simulink model "BD_PAR_AUTO_base_model"  (Simulink 10.3)
settings: Solver=ode1  StartTime=0.0  StopTime=max(cyc_mph(:,1))  FixedStep=1  MaxStep=1  RelTol=1e-3  AbsTol=1e-3
undefined symbols (not defined in the file): acc_dcdc_eff, acc_elec_eff, acc_elec_pwr, acc_mech_eff, acc_mech_pwr, acc_mech_trq, air_cp, amb_tmp, cs_charge_deplete_bool, cs_charge_trq, cs_electric_decel_spd, cs_electric_launch_spd_hi, cs_electric_launch_spd_lo, cs_hi_soc, cs_lo_soc, cs_min_trq_frac, cs_off_trq_frac, cyc_avg_time, cyc_cargo_mass, cyc_elevation_init, cyc_filter_bool, cyc_grade, cyc_mph, enable_sim_stop_distance, enable_sim_stop_max_spd, enable_sim_stop_speed, enable_sim_stop_time, enable_stop, enable_stop_fc, ess_cap_scale, ess_coulombic_eff, ess_init_soc, ess_max_ah_cap, ess_max_volts, ess_min_volts, ess_mod_airflow, ess_mod_cp, ess_mod_init_tmp, ess_module_mass, ess_module_num, ess_on, ess_r_chg, ess_r_dis, ess_res_scale_coef, ess_res_scale_fun, ess_set_tmp, ess_soc, ess_th_calc, ess_th_res_off, ess_th_res_on, ess_tmp, ess_voc, ex_calc, ex_cat_co_frac, ex_cat_ext_cp, ex_cat_ext_emisv, ex_cat_ext_init_tmp, ex_cat_ext_mass, ex_cat_ext_sarea, ex_cat_hc_frac ... (+168)
(part 3 of 15)

== system BD_PAR_AUTO_base_model/<vc> par auto/motor controller logic ==
  bus voltage : Inport
  req'd input power (W) : Inport  Port=2
  req'd output spd (rad/s) : Inport  Port=3
  shifting : Inport  Port=4
  Abs : Abs
  Abs1 : Abs
  Block NOTES : Subsystem
      mask Display: disp('Block\nNOTES')
  Constant : Constant  Value=mc_max_crrnt
  Constant1 : Constant  Value=0.001
  Constant2 : Constant  Value=0
  Logical Operator1 : Logic  Operator=NOT  Inputs=1
  Memory : Memory  InitialCondition=ess_module_num*mean(ess_voc(1,:))
  MinMax : MinMax  Inputs=2  InputSameDT=on  SaturateOnIntegerOverflow=on
  Product1 : Product  InputSameDT=on  RndMeth=Zero  SaturateOnIntegerOverflow=on  OutDataTypeStr=Inherit: Same as first input
  Relational Operator : RelationalOperator  Operator=<=  RndMeth=Nearest  InputSameDT=on
  Relational Operator2 : RelationalOperator  Operator===  RndMeth=Nearest  InputSameDT=on
  Sign : Subsystem  mask(Sign){}
      mask help: y = sign(x)
      mask Help: Sign Function:\n\t\t\ty = 1 if x > 0\n\t\t\ty = 0 if x = 0\n\t\t\ty = -1 if x < 0
      mask Display: plot(-50,-50,50,50,[-50,50],[0,0],[0,0],[-50,50],[-40,0],[-30,-30],[0,40],[30,30])
  Switch : Switch  Threshold=eps
  current-limited power : Product  InputSameDT=on  RndMeth=Zero  SaturateOnIntegerOverflow=on  OutDataTypeStr=Inherit: Same as first input
  true if motor should be shut down : Logic  Operator=OR
  req'd input power (W)1 : Outport  InitialOutput=0
  tag scope: mc_crrnt_limited=global
  wires:
  shifting/1 -> true if motor should be shut down/2
  Logical Operator1/1 -> Switch/2
  true if motor should be shut down/1 -> Logical Operator1/1
  Memory/1 -> Product1/1
  bus voltage/1 -> Memory/1
  Constant/1 -> Product1/2
  req'd input power (W)/1 -> Abs/1, Sign/1(in_1)
  Abs/1 -> MinMax/2
  Sign/1(out_1) -> current-limited power/2
  Constant2/1 -> Switch/3
  Switch/1 -> req'd input power (W)1/1
  current-limited power/1 -> Switch/1
  Product1/1 -> MinMax/1, Relational Operator2/1
  MinMax/1 -> current-limited power/1, Relational Operator2/2
  Relational Operator2/1 -> [mc_crrnt_limited]
  Relational Operator/1 -> true if motor should be shut down/1
  Constant1/1 -> Relational Operator/2
  req'd output spd (rad/s)/1 -> Abs1/1
  Abs1/1 -> Relational Operator/1

== system BD_PAR_AUTO_base_model/<vc> par auto/parallel clutch control ==
  shifting : Inport
  gb_trq_in_r : Inport  Port=2
  gb_spd_in_r : Inport  Port=3
  engine on : Inport  Port=4
  Block NOTES : Subsystem
      mask Display: disp('Block\nNOTES')
  Clock : Clock
  Constant : Constant  Value=1e-3
  Constant1 : Constant  Value=vc_clutch_bool
  Constant2 : Constant  Value=vc_idle_spd
  Constant3 : Constant  Value=1e-3
  Constant4 : Constant  Value=vc_launch_spd
  Constant5 : Constant  Value=2.5
  Constant6 : Constant
  Fcn: 1 if clutch disengaged 2 if clutch slipping 3 if clutch engaged : Fcn  Expr=u[1]+2*u[2]*(1-u[1])*(1-u[3])+3*u[3]*(1-u[1])
  Logical Operator : Logic
  Logical Operator1 : Logic  Operator=OR
  Manual Switch : ManualSwitch
  Memory : Memory  InitialCondition=1+(2*(cyc_mph(1,2)>0))
  Memory1 : Memory  InitialCondition=cyc_mph(1,2)>0
  Memory2 : Memory  InitialCondition=-1
  Mux : Mux  Inputs=3
  Relational Operator : RelationalOperator  Operator=<=  RndMeth=Nearest  InputSameDT=on
  Relational Operator1 : RelationalOperator  Operator=<  RndMeth=Nearest  InputSameDT=on
  Relational Operator2 : RelationalOperator  Operator=>  RndMeth=Nearest  InputSameDT=on
  Relational Operator3 : RelationalOperator  Operator=<  RndMeth=Nearest  InputSameDT=on
  Sum : Sum  Inputs=+-  InputSameDT=on  SaturateOnIntegerOverflow=on  OutDataTypeStr=Inherit: Same as first input
  Switch : Switch  Threshold=eps
  Switch1 : Switch  Threshold=0.5
  Transport Delay : TransportDelay  DelayTime=0.2
  clutch disengaged : Logic  Operator=OR
  clutch engaged : Logic  Operator=NOR
  clutch slipping : Logic  Inputs=3
  clutch slipping1 : Logic
  clutch slipping2 : Logic
  clutch was NOT fully engaged during last time step : RelationalOperator  Operator=<  RndMeth=Nearest  InputSameDT=on
  gearbox speed estimator : Subsystem
  clutch state : Outport
  wires:
  Switch/1 -> Memory/1, clutch state/1
  Fcn: 1 if clutch disengaged 2 if clutch slipping 3 if clutch engaged/1 -> Switch/1
  Manual Switch/1 -> Switch/2
  Switch1/1 -> Manual Switch/2
  gearbox speed estimator/1(Out1) -> Relational Operator3/1, Relational Operator1/1
  gb_spd_in_r/1 -> gearbox speed estimator/1(gb_spd_in_r if no gear change)
  Sum/1 -> Switch1/2
  Memory2/1 -> Sum/2
  Clock/1 -> Memory2/1, Sum/1
  clutch slipping2/1 -> Switch1/3
  Transport Delay/1 -> clutch slipping2/2
  clutch slipping1/1 -> Switch1/1
  Memory1/1 -> clutch slipping1/2
  engine on/1 -> Manual Switch/1, clutch slipping2/1, Transport Delay/1, Memory1/1, clutch slipping1/1
  Relational Operator1/1 -> Logical Operator1/2
  Constant2/1 -> Relational Operator1/2
  Mux/1 -> Fcn: 1 if clutch disengaged 2 if clutch slipping 3 if clutch engaged/1
  clutch engaged/1 -> Mux/3
  clutch disengaged/1 -> clutch engaged/1, Mux/1
  Constant3/1 -> Relational Operator2/2
  Relational Operator2/1 -> clutch slipping/1
  clutch slipping/1 -> clutch engaged/2, Mux/2
  Constant4/1 -> Relational Operator3/2
  Relational Operator3/1 -> clutch slipping/2
  Memory/1 -> clutch was NOT fully engaged during last time step/1
  Constant5/1 -> clutch was NOT fully engaged during last time step/2
  clutch was NOT fully engaged during last time step/1 -> clutch slipping/3
  Constant1/1 -> Logical Operator1/1
  Constant/1 -> Relational Operator/2
  Relational Operator/1 -> Logical Operator/1
  Logical Operator1/1 -> Logical Operator/2
  gb_trq_in_r/1 -> Relational Operator2/1, Relational Operator/1
  Logical Operator/1 -> clutch disengaged/2
  shifting/1 -> clutch disengaged/1
  Constant6/1 -> Switch/3

== system BD_PAR_AUTO_base_model/<vc> par auto/sim stop subsystem ==
  Block NOTES : Subsystem
      mask Display: disp('Block\nNOTES')
  Clock : Clock
  Logical Operator : Logic
  Product{,1..3} (4 alike) : Product  InputSameDT=on  RndMeth=Zero  SaturateOnIntegerOverflow=on  OutDataTypeStr=Inherit: Same as first input
  Relational Operator : RelationalOperator  Operator=>  RndMeth=Nearest  InputSameDT=on
  Relational Operator1 : RelationalOperator  Operator===  RndMeth=Nearest  InputSameDT=on
  Stop Simulation : Stop
  Stop Simulation1 : Stop
  Sum : Sum  Inputs=++++  InputSameDT=on  SaturateOnIntegerOverflow=on  OutDataTypeStr=Inherit: Same as first input
  Sum1 : Sum  Inputs=++++  InputSameDT=on  SaturateOnIntegerOverflow=on  OutDataTypeStr=Inherit: Same as first input
  do ex calcs?2 : Constant  Value=enable_stop_fc
  do ex calcs?3 : Constant  Value=enable_sim_stop_distance
  do ex calcs?4 : Constant  Value=enable_sim_stop_speed
  do ex calcs?5 : Constant  Value=enable_sim_stop_time
  do ex calcs?6 : Constant  Value=enable_sim_stop_max_spd
  do ex calcs?7 : Constant  Value=0
  stop sim distance : Subsystem  TreatAsAtomicUnit=on
  stop sim fc : Subsystem  TreatAsAtomicUnit=on
  stop sim max spd : Subsystem  TreatAsAtomicUnit=on
  stop sim speed : Subsystem  TreatAsAtomicUnit=on
  stop sim time : Subsystem  TreatAsAtomicUnit=on
  wires:
  do ex calcs?2/1 -> stop sim fc/Enable
  [engine_on] -> stop sim fc/1(engine on?)
  [distance] -> stop sim distance/1(distance)
  [mpha] -> stop sim speed/1(speed)
  Clock/1 -> stop sim time/1(time)
  [mpha] -> stop sim max spd/1(speed)
  stop sim distance/1(Out1) -> Product/2
  do ex calcs?3/1 -> stop sim distance/Enable, Product/1, Sum/1
  stop sim max spd/1(Out1) -> Product3/2
  stop sim time/1(Out1) -> Product2/2
  stop sim speed/1(Out1) -> Product1/2
  do ex calcs?4/1 -> stop sim speed/Enable, Product1/1, Sum/2
  do ex calcs?5/1 -> stop sim time/Enable, Product2/1, Sum/3
  do ex calcs?6/1 -> stop sim max spd/Enable, Product3/1, Sum/4
  Product/1 -> Sum1/1
  Product1/1 -> Sum1/2
  Product2/1 -> Sum1/3
  Product3/1 -> Sum1/4
  Logical Operator/1 -> Stop Simulation/1
  Sum1/1 -> Relational Operator1/2
  Sum/1 -> Relational Operator1/1, Relational Operator/1
  do ex calcs?7/1 -> Relational Operator/2
  Relational Operator/1 -> Logical Operator/1
  Relational Operator1/1 -> Logical Operator/2
  stop sim fc/1(Out1) -> Stop Simulation1/1

== system BD_PAR_AUTO_base_model/Interactive Graphics/off ==
  Altia_Run : Constant  Value=0
  tag scope: Altia_Run=global
  wires:
  Altia_Run/1 -> [Altia_Run]

== system BD_PAR_AUTO_base_model/NOTES/NOTES ==
  note: ADVISOR 2.0.2 10/7/98
      | Copyright 1998-2003  MRI, NREL.
      | All rights reserved
      |
      |  Notice:  This computer software was
      |  prepared by NREL/MRI, and hereinafter the Contractor,
      | under Contract No. DE-AC36-83CH10093 with
      | the Department of Energy (DOE).  All rights
      | in the computer software are reserved by DOE
      | on behalf of the United States Government and
      | the Contractor as provided in the contract.
      | You are authorized to use this computer software
      | for Governmental purposes but it is not to be
      | released or distributed to the public.  NEITHER
      | THE GOVERNMENT NOR THE CONTRACTOR MAKES ANY
      | WARRANTY, EXPRESS OR IMPLIED, OR ASSUMES ANY
      | LIABILITY FOR THE USE OF THIS SOFTWARE.
      | This notice including this sentence must
      | appear on any copies of this computer software.

== system BD_PAR_AUTO_base_model/clutch <cl>/help ==

== system BD_PAR_AUTO_base_model/drive cycle <cyc>/Block NOTES ==
  note: This block determines the speed required of the vehicle.  If cyc_filter_bool
      | is true, a centered-in-time average of the trace, with backlash, is required of
      | the vehicle.  This may be useful to smooth out jumps in the trace.  Otherwise,
      | the trace, exactly as published, is required of the vehicle.
      | This block also determines the roadway grade of the cycle and the
      | elevation as a function of the distance travelelled

== system BD_PAR_AUTO_base_model/drive cycle <cyc>/ambient pressure calc (atm) ==
  elevation : Inport
  Gain1 : Gain  Gain=-1  SaturateOnIntegerOverflow=on  OutDataTypeStr=Inherit: Same as input  ParamDataTypeStr=Inherit: Same as input
  Height Scale Factor (1/m) : Constant  Value=1.16546e-4
  Math Function : Math  SignedPower=on
  Product9 : Product  InputSameDT=on  RndMeth=Zero  SaturateOnIntegerOverflow=on  OutDataTypeStr=Inherit: Same as first input
  Out1 : Outport
  wires:
  Math Function/1 -> Out1/1
  Height Scale Factor (1/m)/1 -> Product9/2
  Gain1/1 -> Product9/1
  elevation/1 -> Gain1/1
  Product9/1 -> Math Function/1

== system BD_PAR_AUTO_base_model/drive cycle <cyc>/distance travelled (m) ==
  Block NOTES : Subsystem
      mask Display: disp('Block\nNOTES')
  Integrator : Integrator
  mph-->m/s : Gain  Gain=0.447  SaturateOnIntegerOverflow=on  OutDataTypeStr=Inherit: Same as input  ParamDataTypeStr=Inherit: Same as input
  Out1 : Outport  InitialOutput=0
  wires:
  mph-->m/s/1 -> Integrator/1
  [mpha] -> mph-->m/s/1
  Integrator/1 -> Out1/1

== system BD_PAR_AUTO_base_model/drive cycle <cyc>/repeated cycle grade vs. distance ==
  distance travelled (m) : Inport
  Fcn1 : Fcn  Expr=rem(u[1],period)
  Look-Up Table : Lookup  InputValues=t  Table=y
  out_1 : Outport  InitialOutput=0
  wires:
  Look-Up Table/1 -> out_1/1
  Fcn1/1 -> Look-Up Table/1
  distance travelled (m)/1 -> Fcn1/1

== system BD_PAR_AUTO_base_model/drive cycle <cyc>/repeated cycle speed vs. time ==
  Clock : Clock
  Fcn1 : Fcn  Expr=rem(u[1],period)
  Look-Up Table : Lookup  InputValues=t  Table=y
  out_1 : Outport  InitialOutput=0
  wires:
  Look-Up Table/1 -> out_1/1
  Clock/1 -> Fcn1/1
  Fcn1/1 -> Look-Up Table/1

== system BD_PAR_AUTO_base_model/drive cycle <cyc>/repeated cycle vehicle cargo mass vs. distance ==
  distance travelled (m) : Inport
  Fcn1 : Fcn  Expr=rem(u[1],period)
  Look-Up Table : Lookup  InputValues=t  Table=y
  out_1 : Outport  InitialOutput=0
  wires:
  Look-Up Table/1 -> out_1/1
  Fcn1/1 -> Look-Up Table/1
  distance travelled (m)/1 -> Fcn1/1

== system BD_PAR_AUTO_base_model/drive cycle <cyc>/super-smooth, no-lag trace ==
  Subsystem : Subsystem  mask(Running Average){n=avgtime}
      mask prompts: n "Averaging Time (s)"
      mask help: Running Average
      mask Help: Output is the average of the last (Averaging Time) seconds of input.
      mask Display: disp('Running\nAverage')
  repeated cycle : Subsystem
  out_1 : Outport  InitialOutput=0
  wires:
  repeated cycle/1(out_1) -> Subsystem/1(in_1)
  Subsystem/1(out_1) -> out_1/1

== system BD_PAR_AUTO_base_model/electric acc loads <acc>/Electrical Accessory Loads v2 <acc> ==
  note: Data Logging
  note: Backward-Forward Models
  note: INTERFACE
  "requested electrical Power, out to the driveline (W)" : Inport
  achieved power in from power source (W) : Inport  Port=2
  on/off : Inport  Port=3
  Accessory SDO : Subsystem
  Block NOTES : Subsystem
      mask Display: disp('Block\nNOTES')
  Mux3 : Mux  Inputs=3
  backward model : Subsystem
  forward model : Subsystem
  memory : Memory  InitialCondition=acc_elec_pwr
  "requested electrical Power, in from the power source (W)" : Outport
  "achieved electrical Power, out to the driveline (W)" : Outport  Port=2
  tag scope: acc_elec_pwr_a=global, acc_elec_pwr_est=global, acc_elec_pwr_r=global
  wires:
  [acc_on] -> backward model/2(on/off)
  on/off/1 -> [acc_on]
  memory/1 -> [acc_elec_pwr_est]
  forward model/2(acc_pwr_out) -> memory/1, [acc_elec_pwr_a]
  [acc_elec_pwr_r] -> forward model/2(acc_pwr_in)
  [acc_elec_pwr_est] -> Mux3/3
  [acc_elec_pwr_a] -> Mux3/2
  [acc_elec_pwr_r] -> Mux3/1
  backward model/2(elec_acc_out) -> [acc_elec_pwr_r]
  Mux3/1 -> Accessory SDO/1(data bus)
  forward model/1(pwr_out) -> [driveline_pwr_out_a]
  [powersource_pwr_in_a] -> forward model/1(pwr_in)
  backward model/1(elec_out) -> [powersource_pwr_in_r]
  [driveline_pwr_out_r] -> backward model/1(pwr_in)
  [driveline_pwr_out_a] -> "achieved electrical Power, out to the driveline (W)"/1
  [powersource_pwr_in_r] -> "requested electrical Power, in from the power source (W)"/1
  achieved power in from power source (W)/1 -> [powersource_pwr_in_a]
  "requested electrical Power, out to the driveline (W)"/1 -> [driveline_pwr_out_r]

== system BD_PAR_AUTO_base_model/electric assist control strategy <cs>/chg trq req'd (Nm) ==
  Constant : Constant  Value=cs_charge_trq*fc_trq_scale
  Constant1 : Constant  Value=ess_on
  Goal : Constant  Value=(cs_lo_soc+cs_hi_soc)/2
  Product : Product  InputSameDT=on  RndMeth=Zero  SaturateOnIntegerOverflow=on  OutDataTypeStr=Inherit: Same as first input
  Product1 : Product  Inputs=*/  InputSameDT=on  RndMeth=Zero  SaturateOnIntegerOverflow=on  OutDataTypeStr=Inherit: Same as first input
  Range : Constant  Value=(cs_hi_soc-cs_lo_soc)/2
  Saturation : Saturate  UpperLimit=inf  LowerLimit=-inf
  Sum : Sum  Inputs=-+  InputSameDT=on  SaturateOnIntegerOverflow=on  OutDataTypeStr=Inherit: Same as first input
  Switch : Switch  Threshold=eps
  add'l trq req'd (Nm) : Outport
  wires:
  Constant1/1 -> Switch/3, Switch/2
  Switch/1 -> add'l trq req'd (Nm)/1
  Saturation/1 -> Switch/1
  [SOC] -> Sum/1
  Goal/1 -> Sum/2
  Range/1 -> Product1/2
  Sum/1 -> Product1/1
  Product1/1 -> Product/2
  Constant/1 -> Product/1
  Product/1 -> Saturation/1

== system BD_PAR_AUTO_base_model/electric assist control strategy <cs>/help ==

== system BD_PAR_AUTO_base_model/electric assist control strategy <cs>/minimum trq (Nm) ==
  "trq and spd req'd into trq coupler (N*m, rad/s)" : Inport
  (--) : Constant  Value=cs_lo_soc
  Constant : Constant  Value=0
  Gain : Gain  Gain=cs_min_trq_frac  SaturateOnIntegerOverflow=on  OutDataTypeStr=Inherit: Same as input  ParamDataTypeStr=Inherit: Same as input
  Relational Operator2 : RelationalOperator  Operator=<  RndMeth=Nearest  InputSameDT=on
  Selector : Selector  InputPortWidth=2  IndexOptions=Index vector (dialog)  Indices=2  OutputSizes=1
  Switch : Switch  Threshold=eps
  Terminator : Terminator
  constant threshhold trq (N*m) : Constant  Value=max(fc_max_trq)*0.33
  max_torque lookup : Lookup  InputValues=fc_map_spd  Table=fc_max_trq*fc_trq_scale
  minimum trq (N*m) : Outport
  wires:
  Gain/1 -> Switch/1
  max_torque lookup/1 -> Gain/1
  Selector/1 -> max_torque lookup/1
  "trq and spd req'd into trq coupler (N*m, rad/s)"/1 -> Selector/1
  constant threshhold trq (N*m)/1 -> Terminator/1
  Constant/1 -> Switch/3
  Switch/1 -> minimum trq (N*m)/1
  Relational Operator2/1 -> Switch/2
  (--)/1 -> Relational Operator2/2
  [SOC] -> Relational Operator2/1

== system BD_PAR_AUTO_base_model/energy storage <ess>/ess config ==
  power req'd into bus (W) : Inport
  energy storage <ess> : Subsystem
      mask Display: image(imread('bdi_ess.jpg'))
  power available to bus (W) : Outport
  wires:
  power req'd into bus (W)/1 -> energy storage <ess>/1(power req'd into bus (W))
  energy storage <ess>/1(power available to bus (W)) -> power available to bus (W)/1

== system BD_PAR_AUTO_base_model/exhaust sys <ex>/Block NOTES ==
  note: This block models the exhaust system of an internal combustion engine (ICE).  Emphasis is on the catalytic converter
      | aftertreatment of emissions.  Since converter performance is tied to operating temperature, the temperature and heat
      | flows of the exhaust gas, converter, and engine manifold/downpipe are predicted.

== system BD_PAR_AUTO_base_model/exhaust sys <ex>/ex gas heat flow ==
  emis cat'd : Inport
  ex gas flow : Inport  Port=2
  Tex,eo : Inport  Port=3
  ex_temp : Inport  Port=4
  Enable : EnablePort  StatesWhenEnabling=reset
  % : Gain  Gain=100  SaturateOnIntegerOverflow=on
  %1 : Gain  Gain=669  SaturateOnIntegerOverflow=on
  %2 : Gain  Gain=121  SaturateOnIntegerOverflow=on
  %3 : Gain  Gain=93+79/3  SaturateOnIntegerOverflow=on
  %5 : Gain  Gain=0  SaturateOnIntegerOverflow=on
  (eo-tp)/exg : Product  Inputs=*/  SaturateOnIntegerOverflow=on
  Block NOTES : Subsystem
      mask Display: disp('Block\nNOTES')
  Demux3 : Demux
  Memory : Memory  InitialCondition=[0 0 0 0]
  Mux17 : Mux
  Mux19 : Mux  Inputs=3
  Qcp5 : Sum  Inputs=+-  SaturateOnIntegerOverflow=on
  Saturation1 : Saturate  UpperLimit=1  LowerLimit=0
  converter : Subsystem
  cp,exg : Gain  Gain=ex_gas_cp/1000  SaturateOnIntegerOverflow=on
  dTcat : Sum  Inputs=++++  SaturateOnIntegerOverflow=on
  h,exg : Fcn  Expr=23*((u/10)^0.8)
  inlet pipe : Subsystem
  "manifold " : Subsystem
  mol_EO/s : Gain  Gain=[1/44.1 1/28 1/46 1/44]  SaturateOnIntegerOverflow=on
  mol_ex/s : Gain  Gain=1/29  SaturateOnIntegerOverflow=on
  tailpipe  emis : Product  SaturateOnIntegerOverflow=on
  Tex,gas : Outport  OutputWhenDisabled=reset  InitialOutput=amb_tmp
  Qcat : Outport  Port=2  OutputWhenDisabled=reset  InitialOutput=0
  Qex : Outport  Port=3  OutputWhenDisabled=reset  InitialOutput=0
  wires:
  Memory/1 -> mol_EO/s/1
  emis cat'd/1 -> Memory/1
  ex gas flow/1 -> cp,exg/1, h,exg/1, mol_ex/s/1
  "manifold "/1(Texgo) -> inlet pipe/3(Texgi)
  %2/1 -> dTcat/3
  %3/1 -> dTcat/2
  %1/1 -> dTcat/1
  dTcat/1 -> tailpipe  emis/1
  tailpipe  emis/1 -> Qcat/1
  Mux19/1 -> Tex,gas/1
  Mux17/1 -> Qex/1
  [Tgmo] -> Mux19/3
  [Tgpo] -> Mux19/2
  converter/1(Texgo) -> Mux19/1
  converter/2(Qcm2g) -> Mux17/1
  converter/3(Qci2g) -> Mux17/2
  [Qp2g] -> Mux17/3
  [Qma2g] -> Mux17/4
  %5/1 -> dTcat/4
  inlet pipe/1(Texgo) -> converter/3(Texgi)
  Demux3/2 -> Qcp5/1
  Demux3/3 -> Qcp5/2, %2/1
  Demux3/1 -> %1/1
  Qcp5/1 -> %3/1
  Demux3/4 -> %5/1
  Saturation1/1 -> %/1
  mol_ex/s/1 -> (eo-tp)/exg/2
  mol_EO/s/1 -> (eo-tp)/exg/1
  (eo-tp)/exg/1 -> Saturation1/1
  Tex,eo/1 -> "manifold "/3(Texgi)
  ex_temp/1 -> inlet pipe/4(Tex), converter/4(Tex), "manifold "/4(Tex)
  cp,exg/1 -> inlet pipe/2(Cexg), tailpipe  emis/2, converter/2(Cexg), "manifold "/2(Cexg)
  h,exg/1 -> inlet pipe/1(h,exg), converter/1(h,exg), "manifold "/1(h,exg)
  %/1 -> Demux3/1

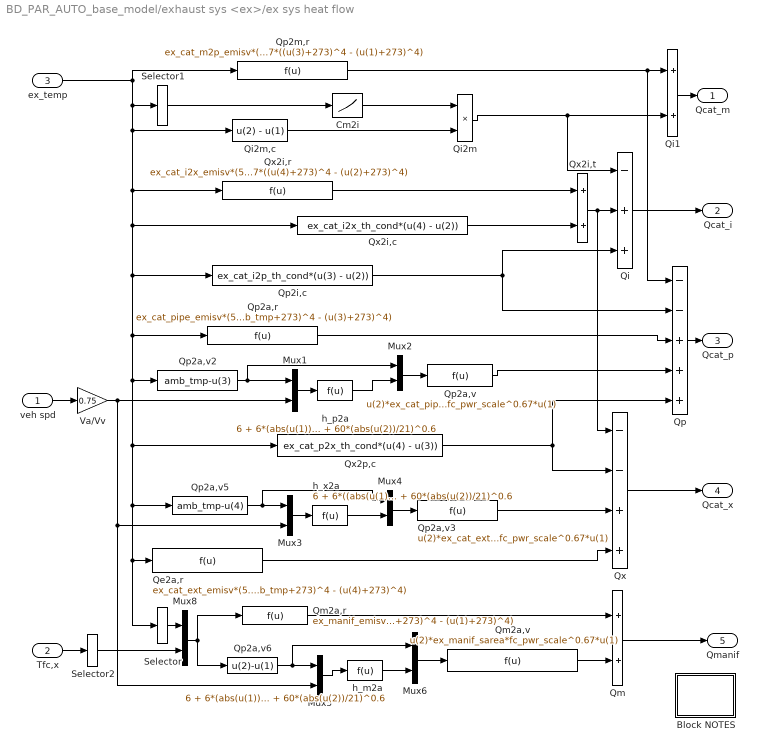
== system BD_PAR_AUTO_base_model/exhaust sys <ex>/ex sys heat flow ==
  veh spd : Inport
  Tfc,x : Inport  Port=2
  ex_temp : Inport  Port=3
  Block NOTES : Subsystem
      mask Display: disp('Block\nNOTES')
  Cm2i : Lookup  InputValues=ex_cat_m2i_tmp  Table=ex_cat_m2i_th_cond
  Mux{1..6,8} (7 alike) : Mux  Inputs=2
  Qe2a,r : Fcn  Expr=ex_cat_ext_emisv*(5.67e-8)*ex_cat_ext_sarea*fc_pwr_scale^0.67*((amb_tmp+273)^4 - (u(4)+273)^4)
  Qi : Sum  Inputs=-++  SaturateOnIntegerOverflow=on
  Qi1 : Sum  SaturateOnIntegerOverflow=on
  Qi2m : Product  SaturateOnIntegerOverflow=on
  Qi2m,c : Fcn  Expr=u(2) - u(1)
  Qm : Sum  SaturateOnIntegerOverflow=on
  Qm2a,r : Fcn  Expr=ex_manif_emisv*(5.67e-8)*ex_manif_sarea*fc_pwr_scale^0.67*((u(2)+273)^4 - (u(1)+273)^4)
  Qm2a,v : Fcn  Expr=u(2)*ex_manif_sarea*fc_pwr_scale^0.67*u(1)
  Qp : Sum  Inputs=--+++  SaturateOnIntegerOverflow=on
  Qp2a,r : Fcn  Expr=ex_cat_pipe_emisv*(5.67e-8)*ex_cat_pipe_sarea*fc_pwr_scale^0.67*((amb_tmp+273)^4 - (u(3)+273)^4)
  Qp2a,v : Fcn  Expr=u(2)*ex_cat_pipe_sarea*fc_pwr_scale^0.67*u(1)
  Qp2a,v2 : Fcn  Expr=amb_tmp-u(3)
  Qp2a,v3 : Fcn  Expr=u(2)*ex_cat_ext_sarea*fc_pwr_scale^0.67*u(1)
  Qp2a,v5 : Fcn  Expr=amb_tmp-u(4)
  Qp2a,v6 : Fcn  Expr=u(2)-u(1)
  Qp2i,c : Fcn  Expr=ex_cat_i2p_th_cond*(u(3) - u(2))
  Qp2m,r : Fcn  Expr=ex_cat_m2p_emisv*(5.67e-8)*ex_cat_monf_sarea*fc_pwr_scale^0.67*((u(3)+273)^4 - (u(1)+273)^4)
  Qx : Sum  Inputs=--++  SaturateOnIntegerOverflow=on
  Qx2i,c : Fcn  Expr=ex_cat_i2x_th_cond*(u(4) - u(2))
  Qx2i,r : Fcn  Expr=ex_cat_i2x_emisv*(5.67e-8)*ex_cat_int_sarea*fc_pwr_scale^0.67*((u(4)+273)^4 - (u(2)+273)^4)
  Qx2i,t : Sum  SaturateOnIntegerOverflow=on
  Qx2p,c : Fcn  Expr=ex_cat_p2x_th_cond*(u(4) - u(3))
  Selector : Selector  InputPortWidth=5  IndexOptions=Index vector (dialog)  Indices=5  OutputSizes=1
  Selector1 : Selector  InputPortWidth=5  IndexOptions=Index vector (dialog)  Indices=[2]  OutputSizes=1
  Selector2 : Selector  InputPortWidth=4  IndexOptions=Index vector (dialog)  Indices=3  OutputSizes=1
  Va/Vv : Gain  Gain=0.75  SaturateOnIntegerOverflow=on
  h_m2a : Fcn  Expr=6 + 6*(abs(u(1))/1000)^0.3 + 60*(abs(u(2))/21)^0.6
  h_p2a : Fcn  Expr=6 + 6*(abs(u(1))/1000)^0.3 + 60*(abs(u(2))/21)^0.6
  h_x2a : Fcn  Expr=6 + 6*((abs(u(1))/1000))^0.3 + 60*(abs(u(2))/21)^0.6
  Qcat_m : Outport
  Qcat_i : Outport  Port=2
  Qcat_p : Outport  Port=3
  Qcat_x : Outport  Port=4
  Qmanif : Outport  Port=5
  wires:
  ex_temp/1 -> Qx2i,c/1, Qx2i,r/1, Qp2m,r/1, Selector1/1, Qi2m,c/1, Qp2i,c/1, Qp2a,r/1, Qp2a,v2/1, Qx2p,c/1, Qp2a,v5/1, Qe2a,r/1, Selector/1
  Qi/1 -> Qcat_i/1
  Qp/1 -> Qcat_p/1
  Mux1/1 -> h_p2a/1
  Qp2a,v2/1 -> Mux1/1, Mux2/1
  Mux4/1 -> Qp2a,v3/1
  Qx/1 -> Qcat_x/1
  Qi1/1 -> Qcat_m/1
  Qx2i,c/1 -> Qx2i,t/2
  Qi2m,c/1 -> Qi2m/2
  Qi2m/1 -> Qi1/2, Qi/1
  Selector1/1 -> Cm2i/1
  Cm2i/1 -> Qi2m/1
  Qp2i,c/1 -> Qi/3, Qp/2
  Qp2m,r/1 -> Qi1/1, Qp/1
  Qp2a,r/1 -> Qp/3
  Qp2a,v/1 -> Qp/4
  Qx2i,r/1 -> Qx2i,t/1
  Qx2i,t/1 -> Qi/2, Qx/1
  Qp2a,v3/1 -> Qx/3
  Mux3/1 -> h_x2a/1
  Qp2a,v5/1 -> Mux3/1, Mux4/1
  h_x2a/1 -> Mux4/2
  Qe2a,r/1 -> Qx/4
  Mux2/1 -> Qp2a,v/1
  h_p2a/1 -> Mux2/2
  Qx2p,c/1 -> Qp/5, Qx/2
  Qm2a,v/1 -> Qm/2
  Qm/1 -> Qmanif/1
  Qm2a,r/1 -> Qm/1
  Mux6/1 -> Qm2a,v/1
  Mux5/1 -> h_m2a/1
  Qp2a,v6/1 -> Mux5/1, Mux6/1
  Selector/1 -> Mux8/1
  Mux8/1 -> Qm2a,r/1, Qp2a,v6/1
  h_m2a/1 -> Mux6/2
  Tfc,x/1 -> Selector2/1
  Selector2/1 -> Mux8/2
  veh spd/1 -> Va/Vv/1
  Va/Vv/1 -> Mux3/2, Mux5/2, Mux1/2

== system BD_PAR_AUTO_base_model/exhaust sys <ex>/help ==

== system BD_PAR_AUTO_base_model/exhaust sys <ex>/removal efficiencies ==
  gas_flow (g/s) : Inport
  Ex Gas T (C) : Inport  Port=2
  O2_exh (g/s) : Inport  Port=3
  emis Engine Out (g/s) : Inport  Port=4
  Ex Cat T (C) : Inport  Port=5
  =1: use ORNL data =0: use base ADVISOR : Constant  Value=ex_ornl_bool
  Switch : Switch  Threshold=eps
  cat in  gas tmp : Selector  InputPortWidth=3  IndexOptions=Index vector (dialog)  Indices=2  OutputSizes=1
  ex_ornl_bool=0 : Logic  Operator=NOT
  removal efficiencies (base ADVISOR) : Subsystem  TreatAsAtomicUnit=on
  removal efficiencies ORNL : Subsystem  TreatAsAtomicUnit=on
  removal effs : Outport  OutputWhenDisabled=reset  InitialOutput=0
  wires:
  removal efficiencies (base ADVISOR)/1(removal effs) -> Switch/1
  removal efficiencies ORNL/1(removal effs) -> Switch/3
  =1: use ORNL data =0: use base ADVISOR/1 -> removal efficiencies ORNL/Enable, ex_ornl_bool=0/1
  O2_exh (g/s)/1 -> removal efficiencies ORNL/3(O2_exh (g/s))
  gas_flow (g/s)/1 -> removal efficiencies ORNL/1(gas_flow (g/s))
  emis Engine Out (g/s)/1 -> removal efficiencies ORNL/4(emis Engine Out (g/s))
  cat in  gas tmp/1 -> removal efficiencies ORNL/2(Ex Gas T (C))
  Ex Gas T (C)/1 -> cat in  gas tmp/1
  Switch/1 -> removal effs/1
  Ex Cat T (C)/1 -> removal efficiencies ORNL/5(Ex Cat T (C)), removal efficiencies (base ADVISOR)/1(Ex Cat T (C))
  ex_ornl_bool=0/1 -> Switch/2, removal efficiencies (base ADVISOR)/Enable

== system BD_PAR_AUTO_base_model/final drive <fd>/Block NOTES ==
  note: The inertia torque is the input torque required to accelerate the
      | final drive's inertia as measured on the input side.
  note: The loss torque is zero when the gears are not turning,
      | and is applied at the input side of the gear reduction.
  note: This final drive model includes loss data, rotational inertia, and a gear reduction.

== system BD_PAR_AUTO_base_model/final drive <fd>/effect of inertia (Nm) ==
  note: The inertia torque is the input torque required to accelerate the
      | final drive's inertia as measured on the input side.
  fd input speed (rad/s) : Inport
  Gain : Gain  Gain=fd_inertia  SaturateOnIntegerOverflow=on
  d/dt : Derivative
  drag torque (Nm) : Outport  InitialOutput=0
  wires:
  fd input speed (rad/s)/1 -> d/dt/1
  d/dt/1 -> Gain/1
  Gain/1 -> drag torque (Nm)/1

== system BD_PAR_AUTO_base_model/final drive <fd>/help ==

== system BD_PAR_AUTO_base_model/final drive <fd>/loss (Nm) ==
  note: The loss torque is zero when the gears are not turning,
      | and is applied at the input side of the gear reduction.
  fd output speed (rad/s) : Inport
  Constant : Constant  Value=0
  Switch : Switch  Threshold=eps
  final drive loss torque (Nm) : Constant  Value=fd_loss
  drag torque (Nm) : Outport  InitialOutput=0
  wires:
  Constant/1 -> Switch/3
  fd output speed (rad/s)/1 -> Switch/2
  Switch/1 -> drag torque (Nm)/1
  final drive loss torque (Nm)/1 -> Switch/1

== system BD_PAR_AUTO_base_model/fuel converter  <fc>/Block NOTES ==
  note: This block models the internal combustion engine, and includes inertia effects,
      | performance limits, accessory loads, and temperature transient effects on fuel
      | use, engine-out emissions, and catalyst efficiency.  There are 'leads' to the
      | engine controller here, which controller determines whether the engine is on.

== system BD_PAR_AUTO_base_model/fuel converter  <fc>/engine controller interface ==
  fc_spd_out_r : Inport
  spd command : Outport
  tag scope: fc_spd_out_r=global
  wires:
  [spd_command] -> spd command/1
  fc_spd_out_r/1 -> [fc_spd_out_r]

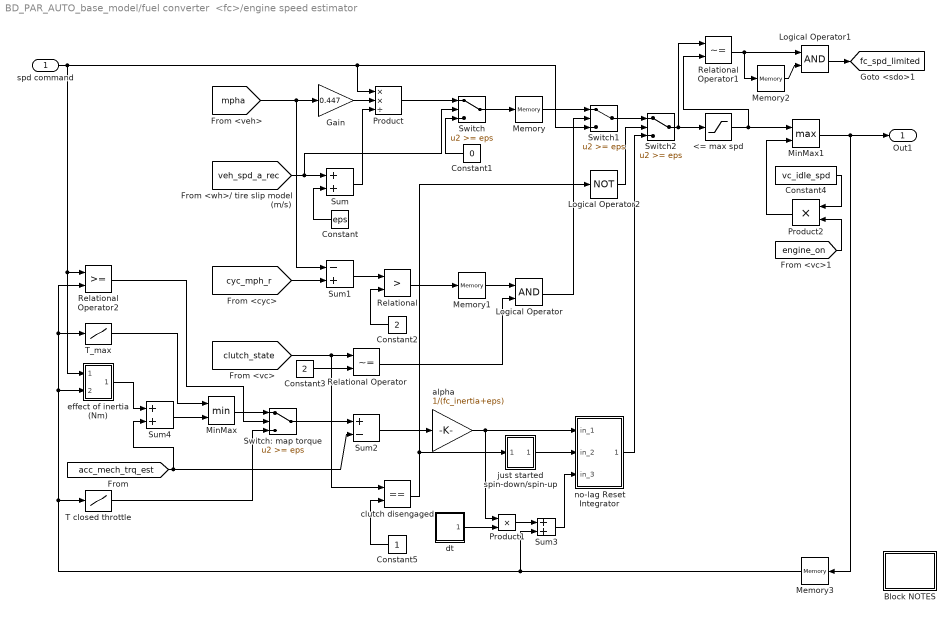
== system BD_PAR_AUTO_base_model/fuel converter  <fc>/engine speed estimator ==
  spd command : Inport
  <= max spd : Saturate  UpperLimit=max(fc_map_spd)*fc_spd_scale  LowerLimit=-inf
  Block NOTES : Subsystem
      mask Display: disp('Block\nNOTES')
  Constant : Constant  Value=eps
  Constant1 : Constant  Value=0
  Constant2 : Constant  Value=2
  Constant3 : Constant  Value=2
  Constant4 : Constant  Value=vc_idle_spd
  Constant5 : Constant
  Gain : Gain  Gain=0.447  SaturateOnIntegerOverflow=on  OutDataTypeStr=Inherit: Same as input  ParamDataTypeStr=Inherit: Same as input
  Logical Operator : Logic
  Logical Operator1 : Logic
  Logical Operator2 : Logic  Operator=NOT  Inputs=1
  Memory : Memory  InitialCondition=cyc_mph(1,2)*0.447/wh_radius*fd_ratio*gb_ratio(gb_num_init)
  Memory1 : Memory
  Memory2 : Memory
  Memory3 : Memory  InitialCondition=cyc_mph(1,2)*0.447/wh_radius*fd_ratio*max(gb_ratio)
  MinMax : MinMax  Inputs=2  InputSameDT=on  SaturateOnIntegerOverflow=on
  MinMax1 : MinMax  Function=max  Inputs=2  InputSameDT=on  SaturateOnIntegerOverflow=on
  Product : Product  Inputs=**/  InputSameDT=on  RndMeth=Zero  SaturateOnIntegerOverflow=on  OutDataTypeStr=Inherit: Same as first input
  Product1 : Product  InputSameDT=on  RndMeth=Zero  SaturateOnIntegerOverflow=on  OutDataTypeStr=Inherit: Same as first input
  Product2 : Product  InputSameDT=on  RndMeth=Zero  SaturateOnIntegerOverflow=on  OutDataTypeStr=Inherit: Same as first input
  Relational : RelationalOperator  Operator=>  RndMeth=Nearest  InputSameDT=on
  Relational Operator : RelationalOperator  Operator=~=  RndMeth=Nearest  InputSameDT=on
  Relational Operator1 : RelationalOperator  Operator=~=  RndMeth=Nearest  InputSameDT=on
  Relational Operator2 : RelationalOperator  RndMeth=Nearest  InputSameDT=on
  Sum : Sum  InputSameDT=on  SaturateOnIntegerOverflow=on  OutDataTypeStr=Inherit: Same as first input
  Sum1 : Sum  Inputs=-+  InputSameDT=on  SaturateOnIntegerOverflow=on  OutDataTypeStr=Inherit: Same as first input
  Sum2 : Sum  Inputs=+-  InputSameDT=on  SaturateOnIntegerOverflow=on  OutDataTypeStr=Inherit: Same as first input
  Sum3 : Sum  InputSameDT=on  SaturateOnIntegerOverflow=on  OutDataTypeStr=Inherit: Same as first input
  Sum4 : Sum  InputSameDT=on  SaturateOnIntegerOverflow=on  OutDataTypeStr=Inherit: Same as first input
  Switch : Switch  Threshold=eps
  Switch1 : Switch  Threshold=eps
  Switch2 : Switch  Threshold=eps
  Switch: map torque : Switch  Threshold=eps
  T closed throttle : Lookup  InputValues=fc_map_spd*fc_spd_scale  Table=fc_ct_trq*fc_trq_scale
  T_max : Lookup  InputValues=fc_map_spd*fc_spd_scale  Table=fc_max_trq*fc_trq_scale
  alpha : Gain  Gain=1/(fc_inertia+eps)  SaturateOnIntegerOverflow=on  OutDataTypeStr=Inherit: Same as input  ParamDataTypeStr=Inherit: Same as input
  clutch disengaged : RelationalOperator  Operator===  RndMeth=Nearest  InputSameDT=on
  dt : Subsystem
  effect of inertia (Nm) : Subsystem
  just started spin-down/spin-up : Subsystem
  no-lag Reset Integrator : Subsystem  mask(No-lag Reset Integrator){initval=vc_idle_spd}
      mask prompts: initval "Initial Value"
      mask help: No-lag Reset Integrator
      mask Help: Integrates first input using Euler technique.\nAt the time step that input 2 <> zero,\noutput is reset to input 3.
      mask Display: disp('1/s\nw/ reset\nno lag')
  Out1 : Outport
  tag scope: fc_spd_limited=global
  wires:
  [acc_mech_trq_est] -> Sum2/2, Sum4/2
  Product/1 -> Switch/1
  [veh_spd_a_rec] -> Sum/1, Switch/2
  Constant1/1 -> Switch/3
  Memory/1 -> Switch1/1
  Constant/1 -> Sum/2
  [cyc_mph_r] -> Sum1/2
  [mpha] -> Gain/1, Sum1/1
  Constant2/1 -> Relational/2
  Sum1/1 -> Relational/1
  Relational/1 -> Memory1/1
  Switch/1 -> Memory/1
  Gain/1 -> Product/2
  Sum/1 -> Product/3
  Relational Operator/1 -> Logical Operator/2
  Memory1/1 -> Logical Operator/1
  Constant3/1 -> Relational Operator/2
  Sum2/1 -> alpha/1
  dt/1(out_1) -> Product1/2
  Product1/1 -> Sum3/1
  alpha/1 -> Product1/1, no-lag Reset Integrator/1(in_1)
  Constant5/1 -> clutch disengaged/2
  Switch1/1 -> Switch2/1
  clutch disengaged/1 -> Logical Operator2/1, just started spin-down/spin-up/1(state)
  [clutch_state] -> Relational Operator/1, clutch disengaged/1
  Memory3/1 -> Sum3/2, Relational Operator2/2, T_max/1, effect of inertia (Nm)/2(prev spd), T closed throttle/1
  <= max spd/1 -> Relational Operator1/2, MinMax1/1
  [engine_on] -> Product2/2
  Constant4/1 -> Product2/1
  MinMax1/1 -> Out1/1, Memory3/1
  Product2/1 -> MinMax1/2
  Switch2/1 -> <= max spd/1, Relational Operator1/1
  Memory2/1 -> Logical Operator1/2
  Logical Operator1/1 -> [fc_spd_limited]
  Relational Operator1/1 -> Logical Operator1/1, Memory2/1
  Switch: map torque/1 -> Sum2/1
  Relational Operator2/1 -> Switch: map torque/2
  T closed throttle/1 -> Switch: map torque/3
  MinMax/1 -> Switch: map torque/1
  T_max/1 -> MinMax/1
  Sum4/1 -> MinMax/2
  effect of inertia (Nm)/1((Nm)) -> Sum4/1
  spd command/1 -> Relational Operator2/1, effect of inertia (Nm)/1(req'd spd (rad/s)), Switch1/3, Product/1
  Logical Operator2/1 -> Switch2/2
  Logical Operator/1 -> Switch1/2
  no-lag Reset Integrator/1(out_1) -> Switch2/3
  just started spin-down/spin-up/1(trigger) -> no-lag Reset Integrator/2(in_2)
  Sum3/1 -> no-lag Reset Integrator/3(in_3)

== system BD_PAR_AUTO_base_model/fuel converter  <fc>/engine torque ==
  fc_trq_out_r : Inport
  spd command : Inport  Port=2
  engine spd : Inport  Port=3
  Block NOTES : Subsystem
      mask Display: disp('Block\nNOTES')
  Constant1 : Constant  Value=0
  Constant3 : Constant
  Logical Operator : Logic  Operator=OR
  MinMax : MinMax  Inputs=2  InputSameDT=on  SaturateOnIntegerOverflow=on
  MinMax1 : MinMax  Function=max  Inputs=2  InputSameDT=on  SaturateOnIntegerOverflow=on
  Sum : Sum  InputSameDT=on  SaturateOnIntegerOverflow=on  OutDataTypeStr=Inherit: Same as first input
  Sum1 : Sum  Inputs=+-  InputSameDT=on  SaturateOnIntegerOverflow=on  OutDataTypeStr=Inherit: Same as first input
  Switch : Switch  Threshold=eps
  Switch1 : Switch  Threshold=eps
  T_closed throttle : Subsystem
  T_max : Subsystem
  clutch not disengaged : RelationalOperator  Operator=~=  RndMeth=Nearest  InputSameDT=on
  effect of inertia (Nm) : Subsystem
  engine commanded not to decelerate : RelationalOperator  Operator=<=  RndMeth=Nearest  InputSameDT=on
  limited : RelationalOperator  Operator=~=  RndMeth=Nearest  InputSameDT=on
  map torque (Nm) : Outport
  torque to shaft (Nm) : Outport  Port=2
  tag scope: fc_trq_limited=global
  wires:
  Constant1/1 -> Switch1/3
  Sum1/1 -> Switch1/1
  Switch1/1 -> torque to shaft (Nm)/1
  [clutch_state] -> clutch not disengaged/1
  Constant3/1 -> clutch not disengaged/2
  engine commanded not to decelerate/1 -> Logical Operator/1
  Sum/1 -> Switch/1
  Logical Operator/1 -> Switch/2
  limited/1 -> [fc_trq_limited]
  MinMax/1 -> MinMax1/1
  T_max/1(T_max) -> MinMax/2
  T_closed throttle/1(T_closed throttle) -> Switch/3, MinMax1/2
  MinMax1/1 -> limited/2, map torque (Nm)/1, Sum1/1
  Switch/1 -> MinMax/1, limited/1
  clutch not disengaged/1 -> Switch1/2, Logical Operator/2
  engine spd/1 -> T_closed throttle/1(w_APU), T_max/1(w_APU), engine commanded not to decelerate/1, effect of inertia (Nm)/1(engine spd (rad/s))
  fc_trq_out_r/1 -> Sum/1
  effect of inertia (Nm)/1((Nm)) -> Sum/2, Sum1/2
  spd command/1 -> engine commanded not to decelerate/2

== system BD_PAR_AUTO_base_model/fuel converter  <fc>/fuel use and EO emis Configurable Subsystem ==
  T (Nm) : Inport
  w (rad/s) : Inport  Port=2
  fuel use and EO emis : Subsystem
  cumulative fuel  use (gal) : Outport
  "FC ON?, EOem, MFex, Tex, O2ex" : Outport  Port=2
  Vv,Tfc : Outport  Port=3
  wires:
  T (Nm)/1 -> fuel use and EO emis/1(T (Nm))
  w (rad/s)/1 -> fuel use and EO emis/2(w (rad/s))
  fuel use and EO emis/1(cumulative fuel  use (gal)) -> cumulative fuel  use (gal)/1
  fuel use and EO emis/2("FC ON?, EOem, MFex, Tex, O2ex") -> "FC ON?, EOem, MFex, Tex, O2ex"/1
  fuel use and EO emis/3(Vv,Tfc) -> Vv,Tfc/1

== system BD_PAR_AUTO_base_model/fuel converter  <fc>/help ==

== system BD_PAR_AUTO_base_model/gearbox <gb>/Block NOTES ==
  note: This is a good assumption, at least for the VW 4-speed manual transaxle of SAE 820741.
      | In the VW transaxle, efficiency is fairly independent of torque and speed at high torques.
  note: Available output torque is estimated assuming that the gearbox efficiency for theavailable input
      | torque andspeed is the same as the gearbox efficiency for the REQUESTED input torque.
  note: The inertia torque is the input torque required to accelerate the
      | final drive's inertia as measured on the input side.
  note: The loss torque is zero when the gears are not turning,
      | and is applied at the input side of the gear reduction.
  note: This gearbox model includes loss data, rotational inertia, and a gear reduction.

== system BD_PAR_AUTO_base_model/gearbox <gb>/Pout/Pin, neglecting inertia ==
  note: Pout/Pin, neglecting inertia, is used to estimate the output torque given the
      | input torque in a very simple forward-facing calculation.
  Tin : Inport
  Tinertia : Inport  Port=2
  Tout : Inport  Port=3
  gear ratio : Inport  Port=4
  Constant1 : Constant  Value=0
  Pout/Pin (neglecting inertia) : Subsystem
      mask Display: disp('/')
  Product : Product  SaturateOnIntegerOverflow=on
  Relational Operator : RelationalOperator  Operator=~=  RndMeth=Nearest  InputSameDT=on
  Saturation : Saturate  UpperLimit=inf  LowerLimit=0
  Switch : Switch  Threshold=eps
  Tin-Tinertia : Sum  Inputs=+-  SaturateOnIntegerOverflow=on
  make division bombproof : Subsystem
  Pout/Pin : Outport  InitialOutput=0
  wires:
  gear ratio/1 -> Product/1
  Product/1 -> Pout/Pin (neglecting inertia)/2(in_2)
  Tout/1 -> Pout/Pin (neglecting inertia)/1(in_1)
  Tin-Tinertia/1 -> Relational Operator/1, make division bombproof/1(Tin-Tinertia)
  Saturation/1 -> Pout/Pin/1
  Switch/1 -> Saturation/1
  Relational Operator/1 -> Switch/2
  Pout/Pin (neglecting inertia)/1(out_1) -> Switch/1
  Tin/1 -> Tin-Tinertia/1
  Tinertia/1 -> Tin-Tinertia/2
  make division bombproof/1(Out1) -> Product/2
  Constant1/1 -> Relational Operator/2, Switch/3

== system BD_PAR_AUTO_base_model/gearbox <gb>/effect of inertia (Nm) ==
  note: The inertia torque is the input torque required to accelerate the
      | gearbox's inertia as measured on the input side.
  gb input speed (rad/s) : Inport
  Gain : Gain  Gain=gb_inertia  SaturateOnIntegerOverflow=on
  d/dt : Derivative
  drag torque (Nm) : Outport  InitialOutput=0
  wires:
  gb input speed (rad/s)/1 -> d/dt/1
  d/dt/1 -> Gain/1
  Gain/1 -> drag torque (Nm)/1

== system BD_PAR_AUTO_base_model/gearbox <gb>/gearbox controller interface ==
  T_gb_out : Inport
  w_gb_out : Inport  Port=2
  eta_gb : Inport  Port=3
  gear_ratio : Outport  InitialOutput=0
  shifting : Outport  Port=2  InitialOutput=0
  tag scope: T_gb_out=global, eta_gb=global, w_gb_out=global
  wires:
  [shifting] -> shifting/1
  T_gb_out/1 -> [T_gb_out]
  w_gb_out/1 -> [w_gb_out]
  eta_gb/1 -> [eta_gb]
  [gear_ratio] -> gear_ratio/1

== system BD_PAR_AUTO_base_model/gearbox <gb>/gearing (Nm), (rad/s) ==
  "output shaft torque and speed  (Nm), (rad/s)" : Inport
  gear ratio : Inport  Port=2
  Demux : Demux  Outputs=2
  Fcn1 : Fcn  Expr=1/u
  Product2 : Product  SaturateOnIntegerOverflow=on
  Product3 : Product  SaturateOnIntegerOverflow=on
  input shaft torque (Nm) : Outport  InitialOutput=0
  input shaft speed (rad/s) : Outport  Port=2  InitialOutput=0
  wires:
  Demux/2 -> Product3/1
  Demux/1 -> Product2/1
  gear ratio/1 -> Product3/2, Fcn1/1
  "output shaft torque and speed  (Nm), (rad/s)"/1 -> Demux/1
  Fcn1/1 -> Product2/2
  Product2/1 -> input shaft torque (Nm)/1
  Product3/1 -> input shaft speed (rad/s)/1

== system BD_PAR_AUTO_base_model/gearbox <gb>/gearing (Nm), (rad/s)1 ==
  input shaft torque (Nm) : Inport
  input shaft speed (rad/s) : Inport  Port=2
  gear ratio : Inport  Port=3
  Fcn1 : Fcn  Expr=1/u
  Product2 : Product  SaturateOnIntegerOverflow=on
  Product3 : Product  SaturateOnIntegerOverflow=on
  output shaft torque (Nm) : Outport  InitialOutput=0
  output shaft speed (rad/s) : Outport  Port=2  InitialOutput=0
  wires:
  input shaft speed (rad/s)/1 -> Product3/2
  input shaft torque (Nm)/1 -> Product2/1
  Product2/1 -> output shaft torque (Nm)/1
  Product3/1 -> output shaft speed (rad/s)/1
  gear ratio/1 -> Fcn1/1, Product2/2
  Fcn1/1 -> Product3/1

== system BD_PAR_AUTO_base_model/gearbox <gb>/help ==

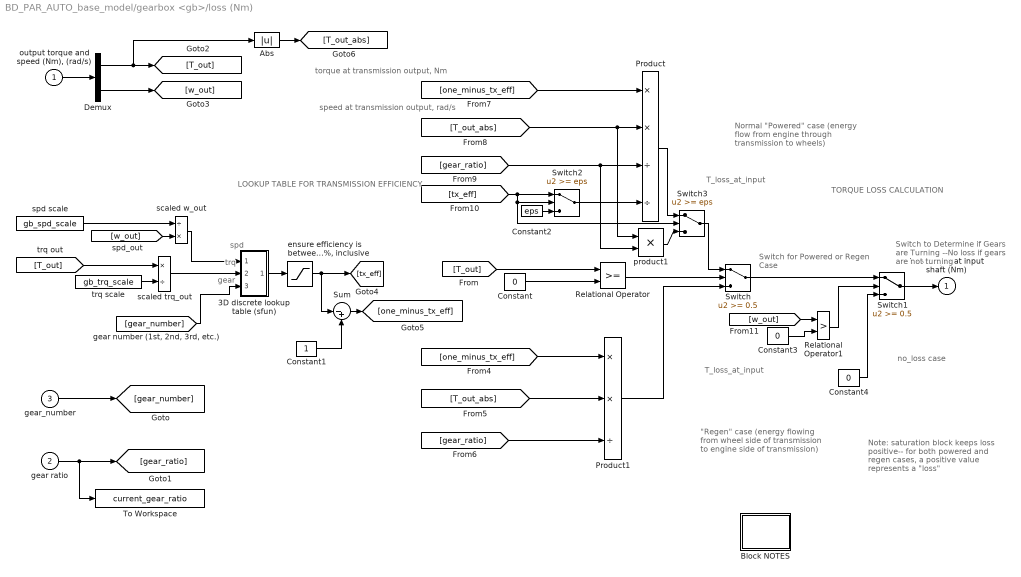
== system BD_PAR_AUTO_base_model/gearbox <gb>/loss (Nm) ==
  note: TORQUE LOSS CALCULATION
  note: gear
  note: trq
  note: spd
  note: torque at transmission output, Nm
  note: speed at transmission output, rad/s
  note: no_loss case
  note: Note: saturation block keeps
      | loss positive-- for both powered
      | and regen cases, a
      | positive value represents a "loss"
  note: Switch for Powered
      |  or Regen Case
  note: Switch to Determine
      | if Gears are Turning
      | --No loss if gears
      | are not turning
  note: Normal "Powered" case
      | (energy flow from engine
      | through transmission to wheels)
  note: T_loss_at_input
  note: "Regen" case
      | (energy flowing from
      | wheel side of transmission
      | to engine side of transmission)
  note: T_loss_at_input
  note: LOOKUP TABLE FOR TRANSMISSION EFFICIENCY
  "output torque and speed (Nm), (rad/s)" : Inport
  gear ratio : Inport  Port=2
  gear_number : Inport  Port=3
  3D discrete lookup table (sfun) : Subsystem  mask{tx_map_spd=tx_map_spd, tx_map_trq=tx_map_trq, tx_eff_map=tx_eff_map}
      mask prompts: tx_map_spd "Row Lookup"; tx_map_trq "Column Lookup"; tx_eff_map "Lookup Matrix"
  Abs : Abs
  Block NOTES : Subsystem
      mask Display: disp('Block\nNOTES')
  Constant : Constant  Value=0
  Constant1 : Constant
  Constant2 : Constant  Value=eps
  Constant3 : Constant  Value=0
  Constant4 : Constant  Value=0
  Demux : Demux  Outputs=2
  Product : Product  Inputs=**//  SaturateOnIntegerOverflow=on
  Product1 : Product  Inputs=**/  SaturateOnIntegerOverflow=on
  Relational Operator : RelationalOperator  RndMeth=Nearest  InputSameDT=on
  Relational Operator1 : RelationalOperator  Operator=>  RndMeth=Nearest  InputSameDT=on
  Sum : Sum  Inputs=|-+  SaturateOnIntegerOverflow=on
  Switch : Switch  Threshold=0.5
  Switch1 : Switch  Threshold=0.5
  Switch2 : Switch  Threshold=eps
  Switch3 : Switch  Threshold=eps
  To Workspace : ToWorkspace  VariableName=current_gear_ratio  SampleTime=-1
      settings: MaxDataPoints=1
  "ensure efficiency is between  0% and 100%, inclusive" : Saturate  UpperLimit=1  LowerLimit=0
  product1 : Product  SaturateOnIntegerOverflow=on
  scaled trq_out : Product  Inputs=*/  SaturateOnIntegerOverflow=on
  scaled w_out : Product  Inputs=/*  SaturateOnIntegerOverflow=on
  spd scale : Constant  Value=gb_spd_scale
  trq scale : Constant  Value=gb_trq_scale
  loss torque at input shaft (Nm) : Outport  InitialOutput=0
  wires:
  product1/1 -> Switch3/3
  Product/1 -> Switch3/1
  Switch3/1 -> Switch/1
  Constant2/1 -> Switch2/3
  [tx_eff] -> Switch3/2, Switch2/2, Switch2/1
  Switch2/1 -> Product/4
  gear_number/1 -> [gear_number]
  gear ratio/1 -> To Workspace/1, [gear_ratio]
  spd scale/1 -> scaled w_out/1
  [w_out] -> scaled w_out/2
  Sum/1 -> [one_minus_tx_eff]
  Constant1/1 -> Sum/2
  trq scale/1 -> scaled trq_out/2
  scaled trq_out/1 -> 3D discrete lookup table (sfun)/2(lookup trq (Nm))
  [T_out] -> scaled trq_out/1
  scaled w_out/1 -> 3D discrete lookup table (sfun)/1(lookup speed (rad/s))
  "ensure efficiency is between  0% and 100%, inclusive"/1 -> Sum/1, [tx_eff]
  3D discrete lookup table (sfun)/1(tx_eff) -> "ensure efficiency is between  0% and 100%, inclusive"/1
  Switch/1 -> Switch1/1
  Abs/1 -> [T_out_abs]
  Demux/1 -> Abs/1, [T_out]
  Relational Operator1/1 -> Switch1/2
  Constant3/1 -> Relational Operator1/2
  [w_out] -> Relational Operator1/1
  Constant4/1 -> Switch1/3
  Switch1/1 -> loss torque at input shaft (Nm)/1
  [gear_ratio] -> product1/2, Product/3
  [T_out_abs] -> product1/1, Product/2
  [one_minus_tx_eff] -> Product/1
  [T_out_abs] -> Product1/2
  [gear_ratio] -> Product1/3
  [one_minus_tx_eff] -> Product1/1
  Product1/1 -> Switch/3
  [T_out] -> Relational Operator/1
  Constant/1 -> Relational Operator/2
  Relational Operator/1 -> Switch/2
  [gear_number] -> 3D discrete lookup table (sfun)/3("gear_number  (e.g., 1, 2, 3)")
  Demux/2 -> [w_out]
  "output torque and speed (Nm), (rad/s)"/1 -> Demux/1

== system BD_PAR_AUTO_base_model/hydraulic torque converter for  parallel hybrid <htc>/Block NOTES ==
  note: This block predicts the relative speed of the HTC input (pump) and output
      | (turbine).  Torque converter lockup is modeled.

== system BD_PAR_AUTO_base_model/hydraulic torque converter for  parallel hybrid <htc>/SR ==
  T,w req out : Inport
  w in : Inport  Port=2
  >0 : Saturate  UpperLimit=inf  LowerLimit=eps
  Constant : Constant  Value=0
  Constant1 : Constant  Value=vc_idle_spd+eps
  Constant3 : Constant
  K_adv : Subsystem
  K_adv_coast : Subsystem
  Logical Operator : Logic  Operator=NOT  Inputs=1
  Logical Operator1 : Logic  Operator=NOT  Inputs=1
  MinMax : MinMax  Inputs=2
  Relational Operator : RelationalOperator  RndMeth=Nearest  InputSameDT=on
  SR Look-Up Table SR=wout/win : Lookup  InputValues=htc_k_adv  Table=htc_sr
  SR Look-Up Table SR=wout/win coast : Lookup  InputValues=fliplr(htc_k_adv_coast)  Table=fliplr(htc_sr_coast)
  SRmax= wout/win,min : Product  Inputs=*/  SaturateOnIntegerOverflow=on
  T : Selector  InputPortWidth=2  IndexOptions=Index vector (dialog)  Indices=1  OutputSizes=1
  To Workspace1 : ToWorkspace  VariableName=htc_locked  SampleTime=-1
  To Workspace3 : ToWorkspace  VariableName=htc_coasting  SampleTime=-1
  if coasting : Switch  Threshold=eps
  "locked up, then SR=1" : Switch  Threshold=eps
  min,max : Saturate  UpperLimit=inf  LowerLimit=1
  shifting SR : Subsystem
  wout,req : Selector  InputPortWidth=2  IndexOptions=Index vector (dialog)  Indices=2  OutputSizes=1
  SR : Outport  InitialOutput=0
  coasting : Outport  Port=2  InitialOutput=0
  wires:
  Relational Operator/1 -> if coasting/2, Logical Operator1/1
  [locked_up] -> To Workspace1/1, Logical Operator/1
  T,w req out/1 -> T/1, K_adv_coast/1("Req'd output trq and spd (Nm), (rad/s)"), wout,req/1, K_adv/1("Req'd output trq and spd (Nm), (rad/s)"), shifting SR/1(T,w req out)
  SR Look-Up Table SR=wout/win coast/1 -> min,max/1
  Constant/1 -> Relational Operator/2
  T/1 -> Relational Operator/1
  Logical Operator/1 -> "locked up, then SR=1"/2
  Constant3/1 -> "locked up, then SR=1"/3
  SR Look-Up Table SR=wout/win/1 -> "locked up, then SR=1"/1
  w in/1 -> shifting SR/2(w in)
  "locked up, then SR=1"/1 -> shifting SR/3(SR)
  shifting SR/1(SR limited) -> if coasting/1
  SRmax= wout/win,min/1 -> MinMax/2
  Constant1/1 -> SRmax= wout/win,min/2
  wout,req/1 -> SRmax= wout/win,min/1
  min,max/1 -> MinMax/1
  MinMax/1 -> if coasting/3
  K_adv_coast/1(K_adv_coast) -> SR Look-Up Table SR=wout/win coast/1
  if coasting/1 -> >0/1
  >0/1 -> SR/1
  Logical Operator1/1 -> To Workspace3/1, coasting/1
  K_adv/1(K_adv) -> SR Look-Up Table SR=wout/win/1

== system BD_PAR_AUTO_base_model/hydraulic torque converter for  parallel hybrid <htc>/T, shifting ==
  TR : Inport
  Req'd  input trq : Inport  Port=2
  Req'd output trq : Inport  Port=3
  htc_spd_in_a : Inport  Port=4
  SR : Inport  Port=5
  Memory : Memory
  Memory1 : Memory
  MinMax : MinMax  Inputs=2
  TR Look-Up Table TR=Tout/Tin : Lookup  InputValues=htc_sr  Table=htc_tr
  T_max : Subsystem
  Tin*TR= Tout,req : Product  SaturateOnIntegerOverflow=on
  engine speed estimator : Subsystem
  "shifting, override zero Trequest" : Switch  Threshold=eps
  T req : Outport
  wires:
  [shifting] -> "shifting, override zero Trequest"/2
  Req'd output trq/1 -> "shifting, override zero Trequest"/3
  htc_spd_in_a/1 -> engine speed estimator/1(htc_spd_in_a)
  SR/1 -> Memory1/1
  Memory1/1 -> TR Look-Up Table TR=Tout/Tin/1
  engine speed estimator/1(Out1) -> T_max/1(w_APU)
  MinMax/1 -> T req/1
  TR Look-Up Table TR=Tout/Tin/1 -> T_max/2(TR)
  "shifting, override zero Trequest"/1 -> MinMax/1
  T_max/1(T_max max gain from htc) -> MinMax/2
  Memory/1 -> "shifting, override zero Trequest"/1
  Req'd  input trq/1 -> Tin*TR= Tout,req/1
  TR/1 -> Tin*TR= Tout,req/2
  Tin*TR= Tout,req/1 -> Memory/1

== system BD_PAR_AUTO_base_model/hydraulic torque converter for  parallel hybrid <htc>/TR ==
  SR : Inport
  coasting : Inport  Port=2
  1/SR*TR  for coast : Fcn  Expr=1/u
  Constant3 : Constant
  Logical Operator : Logic  Operator=NOT  Inputs=1
  Logical Operator1 : Logic  Operator=NOT  Inputs=1
  TR Look-Up Table TR=Tout/Tin : Lookup  InputValues=htc_sr  Table=htc_tr
  TR Look-Up Table TR=Tout/Tin coast : Lookup  InputValues=htc_sr_coast  Table=htc_tr_coast
  To Workspace11 : ToWorkspace  VariableName=htc_efficiency  SampleTime=-1
  effic=SR*TR : Product  Inputs=**  SaturateOnIntegerOverflow=on
  if coasting : Switch  Threshold=eps
  if coasting1 : Switch  Threshold=eps
  "locked up, then TR=1" : Switch  Threshold=eps
  min,max : Saturate  UpperLimit=htc_max_coast_tr  LowerLimit=htc_min_coast_tr
  TR : Outport  InitialOutput=0
  wires:
  TR Look-Up Table TR=Tout/Tin/1 -> "locked up, then TR=1"/1
  Constant3/1 -> "locked up, then TR=1"/3
  [locked_up] -> Logical Operator/1
  Logical Operator/1 -> "locked up, then TR=1"/2
  "locked up, then TR=1"/1 -> if coasting/1
  TR Look-Up Table TR=Tout/Tin coast/1 -> min,max/1
  min,max/1 -> if coasting/3
  SR/1 -> TR Look-Up Table TR=Tout/Tin coast/1, TR Look-Up Table TR=Tout/Tin/1, effic=SR*TR/1
  coasting/1 -> Logical Operator1/1
  if coasting/1 -> TR/1, effic=SR*TR/2
  Logical Operator1/1 -> if coasting/2, if coasting1/2
  effic=SR*TR/1 -> if coasting1/1, 1/SR*TR  for coast/1
  1/SR*TR  for coast/1 -> if coasting1/3
  if coasting1/1 -> To Workspace11/1
